simulink model "Exercise2"  (R2020a)
settings: Solver=VariableStepAuto  StartTime=0.0  StopTime=inf  FixedStep=0.05  RelTol=1e-3
libraries: library_plc2simulink x13
settings Model: EnablePacing=on  Creator=Moritz  LastModifiedBy=Moritz

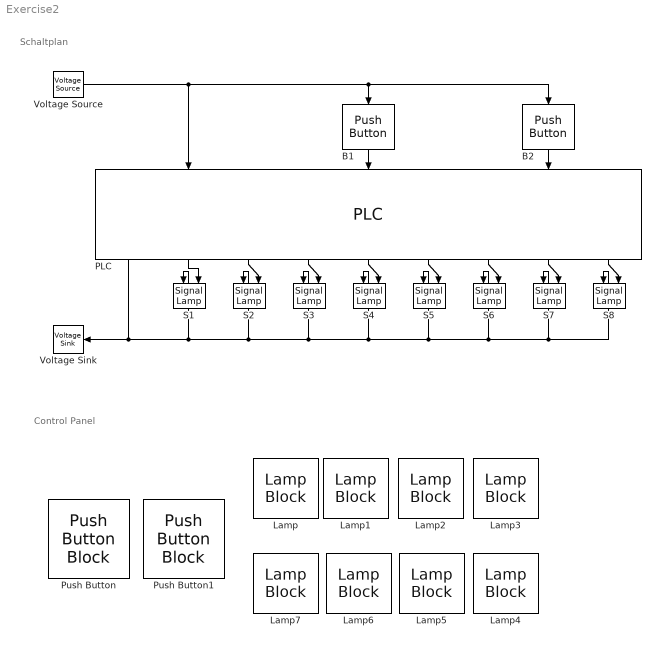
== system Exercise2 ==
  note: Control Panel
  note: Schaltplan
  B1 : library_plc2simulink/Push Button  deactTime=0.3  StateOn=0
  B2 : library_plc2simulink/Push Button  deactTime=0.3  StateOn=0
  Lamp : LampBlock  Tag=S1  LabelPosition=Hide
      settings: AttributesFormatString=S1
  Lamp{1..7} (7 alike) : LampBlock  LabelPosition=Hide
      Lamp1 settings: AttributesFormatString=S2
      Lamp2 settings: AttributesFormatString=S3
      Lamp3 settings: AttributesFormatString=S4
      Lamp4 settings: AttributesFormatString=S5
      Lamp5 settings: AttributesFormatString=S6
      Lamp6 settings: AttributesFormatString=S7
      Lamp7 settings: AttributesFormatString=S8
  PLC : library_plc2simulink/PLC  instanceName=SPSVirtualLab  numInputs=2  numOutputs=8  timeStep=0.05  externalSupplyVoltage=on
  Push Button : PushButtonBlock  ButtonText=B1
  Push Button1 : PushButtonBlock  ButtonText=B2
      settings: AttributesFormatString=B2
  S{1..8} (8 alike) : library_plc2simulink/Signal Lamp  Value=off  updateTime=0.1  colorOn=[0.2,1,0.2]  colorOff=[1,1,1]
  Voltage Sink : library_plc2simulink/Voltage Sink
  Voltage Source : library_plc2simulink/Voltage Source  voltage=24
  wires:
  B1/1 -> PLC/2
  PLC/3 -> S2/1
  PLC/4 -> S3/1
  PLC/6 -> S5/1
  PLC/7 -> S6/1
  PLC/9 -> S8/1
  Voltage Source/1 -> PLC/1, B2/1, B1/1
  PLC/2 -> S1/1
  PLC/5 -> S4/1
  PLC/8 -> S7/1
  B2/1 -> PLC/3
  PLC/1 -> S8/2, S7/2, S6/2, S5/2, S4/2, S3/2, S2/2, S1/2, Voltage Sink/1
